simulink model "DCP"  (R2023a)
settings: Solver=VariableStepAuto  StartTime=0.0  StopTime=4  RelTol=1e-3
model workspace (MAT data in the model file):
  R1 = 20
  R2 = 500
  VT = 0.5
  a = 500
  b = 1000
settings Model: Creator=Wang Xishengshun  LastModifiedBy=Wang Xishengshun

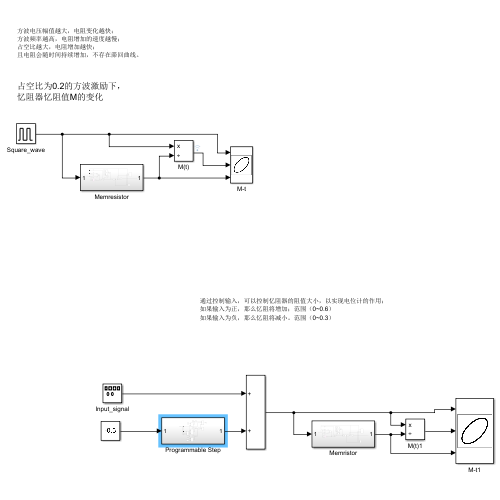
[thumbnail: Simulink's stored preview of the top-level diagram]
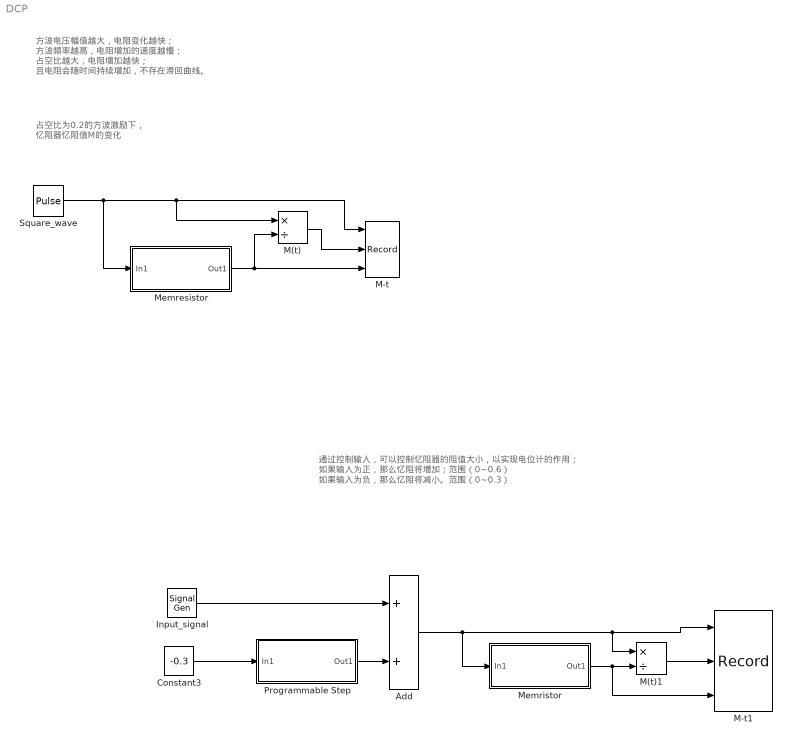
== system DCP ==
  note: 通过控制输入，可以控制忆阻器的阻值大小，以实现电位计的作用；
      | 如果输入为正，那么忆阻将增加；范围（0~0.6）
      | 如果输入为负，那么忆阻将减小。范围（0~0.3）
  note: 占空比为0.2的方波激励下，
      | 忆阻器忆阻值M的变化
  note: 方波电压幅值越大，电阻变化越快；
      | 方波频率越高，电阻增加的速度越慢；
      | 占空比越大，电阻增加越快；
      | 且电阻会随时间持续增加，不存在滞回曲线。
  Add : Sum
  Constant3 : Constant  Value=-0.3
  Input_signal : SignalGenerator  Amplitude=0.1  Frequency=300  Units=rad/sec
  M(t) : Product  Inputs=*/
  M(t)1 : Product  Inputs=*/
  M-t : Record  FileSettingsInternal="{\"entries\":[{\"content\":{\"excelSettings\":{\"content\":{},\"type\":\"Streamout.ExcelSettings\"}},\"type\":\"Streamout.FileSettingStorage\",\"uuid\":\"\"}],\"packageUris\":[\"http:\\/\\/schema.mathworks.com\\/mf0\\/streamout_blocks\\/R2020a\"],\"version\":\"1.0\"}"  Layout=[1 1]  SignalsInternal="{\"entries\":[{\"content\":{\"signals\":[{\"content\":{\"blockPath\":[],\"dimensions\":[1],\"domain\":\"\",\"lineColor\":\"#4dbeee\",\"port\":1,\"signalID\":80,\"signalName\":\"Square_wave\"},\"type\":\"RecordBlkView.Signal\",\"uuid\":\"\"},{\"content\":{\"blockPath\":[],\"dimensions\":[1],\"domain\":\"\",\"lineColor\":\"#a2142f\",\"plots\":[1],\"port\":2,\"signalID\":83,\"signalName\":\"M(t)\"},\"type\":\"RecordBlkView.Signal\",\"uuid\":\"\"},{\"content\":{\"blockPath\":[],\"dimensions\":[1],\"domain\":\"\",\"lineColor\":\"#139fff\",\"port\":3,\"signalID\":86,\"signalName\":\"Memresistor\"},\"type\":\"RecordBlkView.Signal\",\"uuid\":\"\"}]},\"type\":\"RecordBlkView.InputSignals\",\"uuid\":\"\"}],\"packageUris\":[\"http:\\/\\/schema.mathworks.com\\/mf0\\/streamout_blocks\\/R2020a\"],\"version\":\"1.0\"}"  CompatibilityTag=XY
  M-t1 : Record  FileSettingsInternal="{\"entries\":[{\"content\":{\"excelSettings\":{\"content\":{},\"type\":\"Streamout.ExcelSettings\"}},\"type\":\"Streamout.FileSettingStorage\",\"uuid\":\"\"}],\"packageUris\":[\"http:\\/\\/schema.mathworks.com\\/mf0\\/streamout_blocks\\/R2020a\"],\"version\":\"1.0\"}"  Layout=[1 1]  SignalsInternal="{\"entries\":[{\"content\":{\"signals\":[{\"content\":{\"blockPath\":[],\"dimensions\":[1],\"domain\":\"\",\"lineColor\":\"#4dbeee\",\"port\":1,\"signalID\":69,\"signalName\":\"Add\"},\"type\":\"RecordBlkView.Signal\",\"uuid\":\"\"},{\"content\":{\"blockPath\":[],\"dimensions\":[1],\"domain\":\"\",\"lineColor\":\"#a2142f\",\"plots\":[1],\"port\":2,\"signalID\":72,\"signalName\":\"M(t)1\"},\"type\":\"RecordBlkView.Signal\",\"uuid\":\"\"},{\"content\":{\"blockPath\":[],\"dimensions\":[1],\"domain\":\"\",\"lineColor\":\"#139fff\",\"port\":3,\"signalID\":75,\"signalName\":\"Memresistor1\"},\"type\":\"RecordBlkView.Signal\",\"uuid\":\"\"}]},\"type\":\"RecordBlkView.InputSignals\",\"uuid\":\"\"}],\"packageUris\":[\"http:\\/\\/schema.mathworks.com\\/mf0\\/streamout_blocks\\/R2020a\"],\"version\":\"1.0\"}"  VisualizationBindings="{\"sparklinesplugin\":{\"info\":[{\"bindingParametersList\":[],\"subplotID\":1}]}}"  CompatibilityTag=XY
  Memresistor : Subsystem
  Memristor : Subsystem
  Programmable Step : Subsystem
  Square_wave : DiscretePulseGenerator  PulseType=Time based  Amplitude=0.5  Period=1
  wires:
  Add/1 -> M-t1/1, M(t)1/1, Memristor/1(In1)
  M(t)/1 -> M-t/2
  Input_signal/1 -> Add/1
  Constant3/1 -> Programmable Step/1(In1)
  Square_wave/1 -> M(t)/1, M-t/1, Memresistor/1(In1)
  Memresistor/1(Out1) -> M-t/3, M(t)/2
  Programmable Step/1(Out1) -> Add/2
  Memristor/1(Out1) -> M-t1/3, M(t)1/2
  M(t)1/1 -> M-t1/2

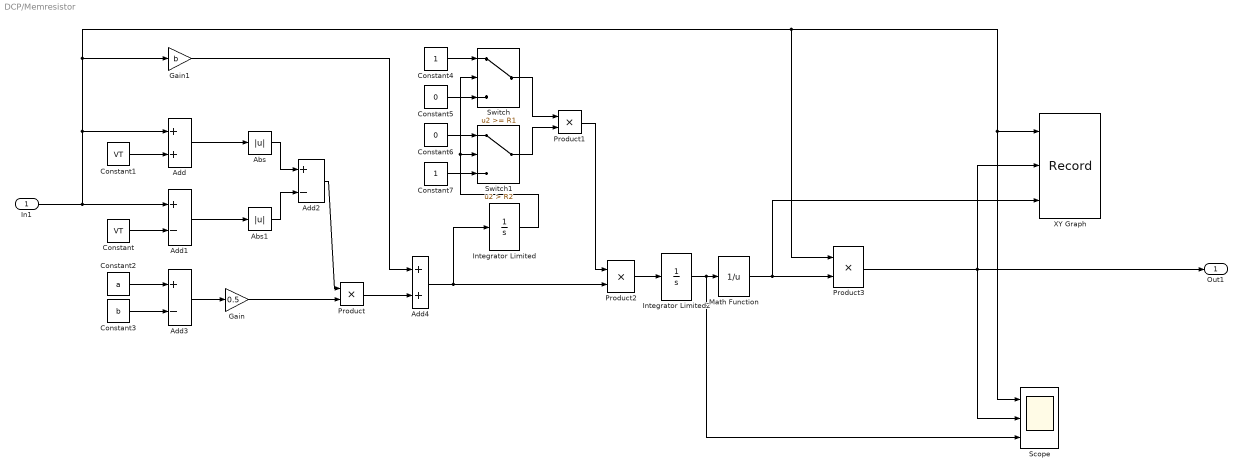
== system DCP/Memresistor ==
  In1 : Inport
  Abs : Abs  SaturateOnIntegerOverflow=off
  Abs1 : Abs  SaturateOnIntegerOverflow=off
  Add : Sum
  Add1 : Sum  Inputs=+-
  Add2 : Sum  Inputs=+-
  Add3 : Sum  Inputs=+-
  Add4 : Sum
  Constant : Constant  Value=VT
  Constant1 : Constant  Value=VT
  Constant2 : Constant  Value=a
  Constant3 : Constant  Value=b
  Constant4 : Constant  SampleTime=0.001
  Constant5 : Constant  Value=0  SampleTime=0.001
  Constant6 : Constant  Value=0  SampleTime=0.001
  Constant7 : Constant  SampleTime=0.001
  Gain : Gain  Gain=0.5
  Gain1 : Gain  Gain=b
  Integrator Limited : Integrator  UpperSaturationLimit=1600  LowerSaturationLimit=0  WrappedStateUpperValue=500  WrappedStateLowerValue=0
  Integrator Limited2 : Integrator  InitialCondition=480  UpperSaturationLimit=1600  LowerSaturationLimit=0  WrappedStateUpperValue=500  WrappedStateLowerValue=0
  Math Function : Math  Operator=reciprocal
  Product{,1..3} (4 alike) : Product
  Scope : Scope  NumInputPorts=3
  Switch : Switch  Threshold=R1  RndMeth=Ceiling  SaturateOnIntegerOverflow=off  InputSameDT=off
  Switch1 : Switch  Criteria=u2 > Threshold  Threshold=R2  RndMeth=Ceiling  SaturateOnIntegerOverflow=off  InputSameDT=off
  XY Graph : Record  FileSettingsInternal="{\"entries\":[{\"content\":{\"excelSettings\":{\"content\":{},\"type\":\"Streamout.ExcelSettings\"}},\"type\":\"Streamout.FileSettingStorage\",\"uuid\":\"\"}],\"packageUris\":[\"http:\\/\\/schema.mathworks.com\\/mf0\\/streamout_blocks\\/R2020a\"],\"version\":\"1.0\"}"  Layout=[2 2]  SignalsInternal="{\"entries\":[{\"content\":{\"signals\":[{\"content\":{\"blockPath\":[],\"dimensions\":[1],\"domain\":\"\",\"lineColor\":\"#7e2f8e\",\"port\":1,\"signalID\":47,\"signalName\":\"In1\"},\"type\":\"RecordBlkView.Signal\",\"uuid\":\"\"},{\"content\":{\"blockPath\":[],\"dimensions\":[1],\"domain\":\"\",\"lineColor\":\"#77ac30\",\"port\":2,\"signalID\":50,\"signalName\":\"Product3\"},\"type\":\"RecordBlkView.Signal\",\"uuid\":\"\"},{\"content\":{\"blockPath\":[],\"dimensions\":[1],\"domain\":\"\",\"lineColor\":\"#4dbeee\",\"port\":3,\"signalID\":53,\"signalName\":\"Math\\nFunction\"},\"type\":\"RecordBlkView.Signal\",\"uuid\":\"\"}]},\"type\":\"RecordBlkView.InputSignals\",\"uuid\":\"\"}],\"packageUris\":[\"http:\\/\\/schema.mathworks.com\\/mf0\\/streamout_blocks\\/R2020a\"],\"version\":\"1.0\"}"  VisualizationBindings="{\"xyplotplugin\":{\"info\":[{\"series\":[],\"subplotID\":1},{\"series\":[],\"subplotID\":9}]}}"  CompatibilityTag=XY
  Out1 : Outport
  wires:
  Product3/1 -> Scope/2, Out1/1, XY Graph/2
  Constant2/1 -> Add3/1
  Product/1 -> Add4/2
  Integrator Limited/1 -> Switch/2, Switch1/2
  Product1/1 -> Product2/1
  Add/1 -> Abs/1
  Math Function/1 -> XY Graph/3, Product3/2
  Gain1/1 -> Add4/1
  Constant7/1 -> Switch1/3
  Constant3/1 -> Add3/2
  Add1/1 -> Abs1/1
  Switch/1 -> Product1/1
  Constant6/1 -> Switch1/1
  Constant5/1 -> Switch/3
  Abs/1 -> Add2/1
  Switch1/1 -> Product1/2
  Product2/1 -> Integrator Limited2/1
  Gain/1 -> Product/2
  Add2/1 -> Product/1
  Constant1/1 -> Add/2
  Constant4/1 -> Switch/1
  Add4/1 -> Integrator Limited/1, Product2/2
  In1/1 -> Add1/1, Scope/1, XY Graph/1, Product3/1, Gain1/1, Add/1
  Integrator Limited2/1 -> Scope/3, Math Function/1
  Abs1/1 -> Add2/2
  Constant/1 -> Add1/2
  Add3/1 -> Gain/1

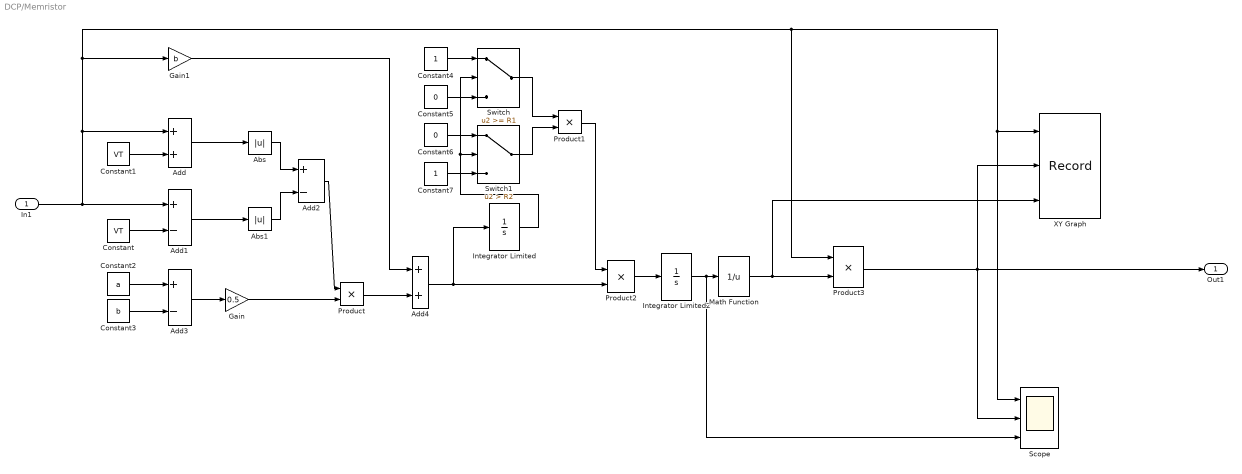
== system DCP/Memristor ==
  In1 : Inport
  Abs : Abs  SaturateOnIntegerOverflow=off
  Abs1 : Abs  SaturateOnIntegerOverflow=off
  Add : Sum
  Add1 : Sum  Inputs=+-
  Add2 : Sum  Inputs=+-
  Add3 : Sum  Inputs=+-
  Add4 : Sum
  Constant : Constant  Value=VT
  Constant1 : Constant  Value=VT
  Constant2 : Constant  Value=a
  Constant3 : Constant  Value=b
  Constant4 : Constant  SampleTime=0.001
  Constant5 : Constant  Value=0  SampleTime=0.001
  Constant6 : Constant  Value=0  SampleTime=0.001
  Constant7 : Constant  SampleTime=0.001
  Gain : Gain  Gain=0.5
  Gain1 : Gain  Gain=b
  Integrator Limited : Integrator  UpperSaturationLimit=1600  LowerSaturationLimit=0  WrappedStateUpperValue=500  WrappedStateLowerValue=0
  Integrator Limited2 : Integrator  InitialCondition=480  UpperSaturationLimit=1600  LowerSaturationLimit=0  WrappedStateUpperValue=500  WrappedStateLowerValue=0
  Math Function : Math  Operator=reciprocal
  Product{,1..3} (4 alike) : Product
  Scope : Scope  NumInputPorts=3
  Switch : Switch  Threshold=R1  RndMeth=Ceiling  SaturateOnIntegerOverflow=off  InputSameDT=off
  Switch1 : Switch  Criteria=u2 > Threshold  Threshold=R2  RndMeth=Ceiling  SaturateOnIntegerOverflow=off  InputSameDT=off
  XY Graph : Record  FileSettingsInternal="{\"entries\":[{\"content\":{\"excelSettings\":{\"content\":{},\"type\":\"Streamout.ExcelSettings\"}},\"type\":\"Streamout.FileSettingStorage\",\"uuid\":\"\"}],\"packageUris\":[\"http:\\/\\/schema.mathworks.com\\/mf0\\/streamout_blocks\\/R2020a\"],\"version\":\"1.0\"}"  Layout=[2 2]  SignalsInternal="{\"entries\":[{\"content\":{\"signals\":[{\"content\":{\"blockPath\":[],\"dimensions\":[1],\"domain\":\"\",\"lineColor\":\"#139fff\",\"port\":1,\"signalID\":58,\"signalName\":\"In1\"},\"type\":\"RecordBlkView.Signal\",\"uuid\":\"\"},{\"content\":{\"blockPath\":[],\"dimensions\":[1],\"domain\":\"\",\"lineColor\":\"#ff6929\",\"port\":2,\"signalID\":61,\"signalName\":\"Product3\"},\"type\":\"RecordBlkView.Signal\",\"uuid\":\"\"},{\"content\":{\"blockPath\":[],\"dimensions\":[1],\"domain\":\"\",\"lineColor\":\"#b746ff\",\"port\":3,\"signalID\":64,\"signalName\":\"Math\\nFunction\"},\"type\":\"RecordBlkView.Signal\",\"uuid\":\"\"}]},\"type\":\"RecordBlkView.InputSignals\",\"uuid\":\"\"}],\"packageUris\":[\"http:\\/\\/schema.mathworks.com\\/mf0\\/streamout_blocks\\/R2020a\"],\"version\":\"1.0\"}"  VisualizationBindings="{\"xyplotplugin\":{\"info\":[{\"series\":[],\"subplotID\":1},{\"series\":[],\"subplotID\":9}]}}"  CompatibilityTag=XY
  Out1 : Outport
  wires:
  Product3/1 -> Scope/2, Out1/1, XY Graph/2
  Constant2/1 -> Add3/1
  Product/1 -> Add4/2
  Integrator Limited/1 -> Switch/2, Switch1/2
  Product1/1 -> Product2/1
  Add/1 -> Abs/1
  Math Function/1 -> XY Graph/3, Product3/2
  Gain1/1 -> Add4/1
  Constant7/1 -> Switch1/3
  Constant3/1 -> Add3/2
  Add1/1 -> Abs1/1
  Switch/1 -> Product1/1
  Constant6/1 -> Switch1/1
  Constant5/1 -> Switch/3
  Abs/1 -> Add2/1
  Switch1/1 -> Product1/2
  Product2/1 -> Integrator Limited2/1
  Gain/1 -> Product/2
  Add2/1 -> Product/1
  Constant1/1 -> Add/2
  Constant4/1 -> Switch/1
  Add4/1 -> Integrator Limited/1, Product2/2
  In1/1 -> Add1/1, Scope/1, XY Graph/1, Product3/1, Gain1/1, Add/1
  Integrator Limited2/1 -> Scope/3, Math Function/1
  Abs1/1 -> Add2/2
  Constant/1 -> Add1/2
  Add3/1 -> Gain/1

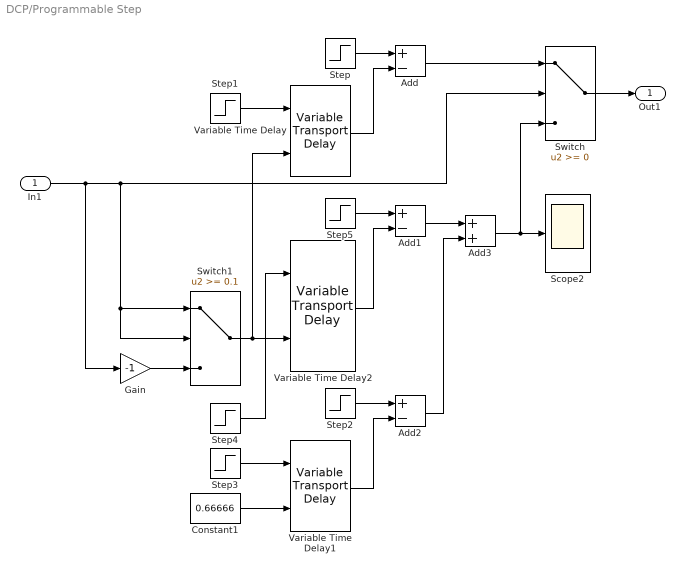
== system DCP/Programmable Step ==
  In1 : Inport
  Add : Sum  Inputs=+-
  Add1 : Sum  Inputs=+-
  Add2 : Sum  Inputs=+-
  Add3 : Sum
  Constant1 : Constant  Value=0.66666
  Gain : Gain  Gain=-1
  Scope2 : Scope
  Step{,1..3} (4 alike) : Step  Time=0  SampleTime=0
  Step4 : Step  After=-1  SampleTime=0
  Step5 : Step  Time=0.66666  After=-1  SampleTime=0
  Switch : Switch  SaturateOnIntegerOverflow=off  InputSameDT=off
  Switch1 : Switch  Threshold=0.1  SaturateOnIntegerOverflow=off  InputSameDT=off
  Variable Time Delay : VariableTransportDelay  MaximumDelay=10  MaximumPoints=3072  ZeroDelay=on
  Variable Time Delay1 : VariableTransportDelay  MaximumDelay=10  MaximumPoints=3072  ZeroDelay=on
  Variable Time Delay2 : VariableTransportDelay  MaximumDelay=10  MaximumPoints=3072  ZeroDelay=on
  Out1 : Outport
  wires:
  In1/1 -> Switch1/2, Switch1/1, Switch/2, Gain/1
  Step5/1 -> Add1/1
  Constant1/1 -> Variable Time Delay1/2
  Variable Time Delay/1 -> Add/2
  Step3/1 -> Variable Time Delay1/1
  Step4/1 -> Variable Time Delay2/1
  Step2/1 -> Add2/1
  Switch1/1 -> Variable Time Delay2/2, Variable Time Delay/2
  Step1/1 -> Variable Time Delay/1
  Switch/1 -> Out1/1
  Gain/1 -> Switch1/3
  Step/1 -> Add/1
  Variable Time Delay2/1 -> Add1/2
  Variable Time Delay1/1 -> Add2/2
  Add/1 -> Switch/1
  Add1/1 -> Add3/1
  Add2/1 -> Add3/2
  Add3/1 -> Switch/3, Scope2/1
